simulink model "RefGen"  (R2018b)
settings: Solver=FixedStepAuto  StartTime=0.0  StopTime=Tsim +Ts*Np  FixedStep=Ts  RelTol=1e-3
values from neighbouring files (symbols this model uses):
  Aref = 8    [simulation.m]    (also in simulationKoop.m)
  fref = 0.7    [simulation.m]    (also in simulationKoop.m)
  Tdref = 0.5    [simulation.m]    (also in simulationKoop.m)
  Tref = 4    [simulation.m]    (also in simulationKoop.m = 3)
  Ts = 0.01    [simulation.m]    (also in simulationKoop.m)
  vehicle = LoadVehicleParameters()    [BicycleModel.m]    (also in TransformInputs.m; mpcController.m; mpcControllerKoop.m; simulation.m)
libraries: simulink_extras x1
settings Model: Creator=Marko  LastModifiedBy=Marko

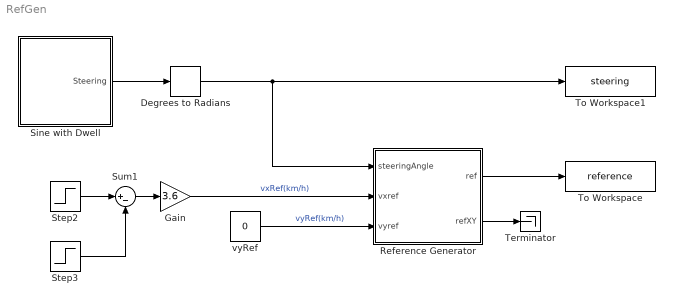
== system RefGen ==
  Degrees to Radians : simulink_extras/Transformations/Degrees to Radians
  Gain : Gain  Gain=3.6
  Reference Generator : Subsystem
  Sine with Dwell : Subsystem
  Step2 : Step  Time=0  After=45/3.6  SampleTime=0
  Step3 : Step  Time=6  After=-35/3.6  SampleTime=0
  Sum1 : Sum  Inputs=|+-
  Terminator : Terminator
  To Workspace : ToWorkspace  VariableName=reference  SaveFormat=Structure With Time  SampleTime=Ts
  To Workspace1 : ToWorkspace  VariableName=steering  SaveFormat=Structure With Time  SampleTime=Ts
  vyRef : Constant  Value=0
  wires:
  Sine with Dwell/1(Steering) -> Degrees to Radians/1
  Sum1/1 -> Gain/1
  Step2/1 -> Sum1/1
  vyRef/1 -> Reference Generator/3(vyref)  "vyRef(km/h)"
  Reference Generator/2(refXY) -> Terminator/1
  Gain/1 -> Reference Generator/2(vxref)  "vxRef(km/h)"
  Step3/1 -> Sum1/2
  Reference Generator/1(ref) -> To Workspace/1
  Degrees to Radians/1 -> Reference Generator/1(steeringAngle), To Workspace1/1

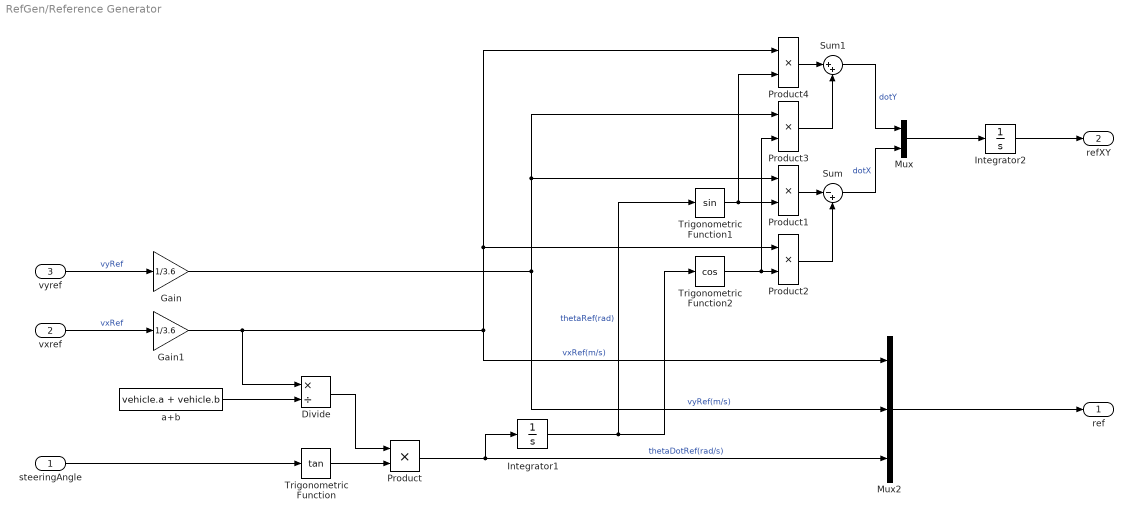
== system RefGen/Reference Generator ==
  steeringAngle : Inport
  vxref : Inport  Port=2
  vyref : Inport  Port=3
  Divide : Product  Inputs=*/
  Gain : Gain  Gain=1/3.6
  Gain1 : Gain  Gain=1/3.6
  Integrator1 : Integrator
  Integrator2 : Integrator  InitialCondition=[0;0]
  Mux : Mux  Inputs=2
  Mux2 : Mux  Inputs=3
  Product{,1..4} (5 alike) : Product
  Sum : Sum  Inputs=|-+
  Sum1 : Sum  Inputs=|++
  Trigonometric Function : Trigonometry  Operator=tan  OutputSignalType=real
  Trigonometric Function1 : Trigonometry
  Trigonometric Function2 : Trigonometry  Operator=cos
  a+b : Constant  Value=vehicle.a + vehicle.b
  ref : Outport
  refXY : Outport  Port=2
  wires:
  a+b/1 -> Divide/2
  vxref/1 -> Gain1/1  "vxRef"
  Product/1 -> Mux2/3, Integrator1/1  "thetaDotRef(rad/s)"
  Divide/1 -> Product/1
  Trigonometric Function/1 -> Product/2
  steeringAngle/1 -> Trigonometric Function/1
  Mux2/1 -> ref/1
  Integrator1/1 -> Trigonometric Function1/1, Trigonometric Function2/1  "thetaRef(rad)"
  Trigonometric Function1/1 -> Product4/2, Product1/2
  Trigonometric Function2/1 -> Product3/2, Product2/2
  Product1/1 -> Sum/1
  Product2/1 -> Sum/2
  Product4/1 -> Sum1/1
  Product3/1 -> Sum1/2
  Sum1/1 -> Mux/1  "dotY"
  Sum/1 -> Mux/2  "dotX"
  Mux/1 -> Integrator2/1
  Integrator2/1 -> refXY/1
  vyref/1 -> Gain/1  "vyRef"
  Gain/1 -> Mux2/2, Product3/1, Product1/1  "vyRef(m/s)"
  Gain1/1 -> Product4/1, Product2/1, Mux2/1, Divide/1  "vxRef(m/s)"

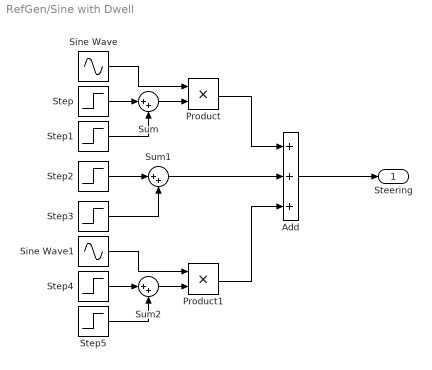
== system RefGen/Sine with Dwell ==
  Add : Sum  Inputs=+++
  Product : Product
  Product1 : Product
  Sine Wave : Sin  Amplitude=Aref  Frequency=2*pi*fref  Phase=-2*pi*fref*Tref  SampleTime=0
  Sine Wave1 : Sin  Amplitude=Aref  Frequency=2*pi*fref  Phase=-2*pi*fref*(Tref+Tdref)  SampleTime=0
  Step : Step  Time=Tref  SampleTime=0
  Step1 : Step  Time=Tref+0.75/fref  After=-1  SampleTime=0
  Step2 : Step  Time=Tref+0.75/fref  After=-Aref  SampleTime=0
  Step3 : Step  Time=Tref+0.75/fref+Tdref  After=Aref  SampleTime=0
  Step4 : Step  Time=Tref+0.75/fref+Tdref  SampleTime=0
  Step5 : Step  Time=Tref+1/fref+Tdref  After=-1  SampleTime=0
  Sum : Sum  Inputs=|++
  Sum1 : Sum  Inputs=|++
  Sum2 : Sum  Inputs=|++
  Steering : Outport
  wires:
  Step2/1 -> Sum1/1
  Sine Wave/1 -> Product/1
  Add/1 -> Steering/1
  Sum1/1 -> Add/2
  Step3/1 -> Sum1/2
  Sum2/1 -> Product1/2
  Product1/1 -> Add/3
  Sine Wave1/1 -> Product1/1
  Step1/1 -> Sum/2
  Step/1 -> Sum/1
  Product/1 -> Add/1
  Step4/1 -> Sum2/1
  Step5/1 -> Sum2/2
  Sum/1 -> Product/2
